simulink model "CF016A_GmVehSpdArbn"  (R2013b)
settings: Solver=FixedStepDiscrete  SolverMode=SingleTasking  StartTime=0.0  StopTime=1  FixedStep=0.002  RelTol=1e-3
undefined symbols (not defined in the file): DIAGCSTRTUPDLY_CNT_U32, NODEBSTEP_CNT_U16, NtcNr1, NtcSts1, VEHSPDMAX_KPH_F32
libraries: simulink x8, NxtrMax x7, NxtrMin x3, NxtrLim x3
(part 5 of 5)

== system CF016A_GmVehSpdArbn/GmVehSpdArbn/GmVehSpdArbnPer1/LeDrvnVld/Set_LeDrvnVld_False ==
  Action Port : ActionPort  ActionType=then
  Constant2 : Constant  Value=false  OutDataTypeStr=boolean
      settings: AttributesFormatString=%<OutDataTypeStr>
  CopyRight2 : Subsystem  Description=|  mask(Copyright Information){none=on}
      | Copyright info block.                                               
      |                                                                     
      | Place copyright information at the top of every subsystem in design.
      mask prompts: none "No parameters"
      mask help: Place copyright information at the top of every subsystem in design.
      mask Display:
      | NxtrConf = 'Nexteer Confidential';
      | 
      | sys = bdroot; %handle for the current model ("system")
      | first = get_param(sys,'Created');
      | if(isempty(first))
      |     first = datestr(now,'yyyy');
      | else
      |     first = first(end-3:end);  %year is last four digits
      | end
      | 
      | last = get_param(sys,'LastModifiedDate');
      | if isempty(last)
      |     last = datestr(now,'yyyy');
      | else
      |     last = last(end-3:end);
      | end
      | 
      | if strcmp(first,last)
      |     fprintf('%s -- Copyright %s Nexteer',NxtrConf,first)
      | else
      |     fprintf('%s -- %s%s- %s Nexteer',NxtrConf,char(169),first,last)
      | end
  LeDrvnVld : Outport
  wires:
  Constant2/1 -> LeDrvnVld/1

== system CF016A_GmVehSpdArbn/GmVehSpdArbn/GmVehSpdArbnPer1/LeDrvnVld/Set_LeDrvnVld_True ==
  Action Port : ActionPort  ActionType=else
  Constant2 : Constant  Value=true  OutDataTypeStr=boolean
      settings: AttributesFormatString=%<OutDataTypeStr>
  CopyRight2 : Subsystem  Description=|  mask(Copyright Information){none=on}
      | Copyright info block.                                               
      |                                                                     
      | Place copyright information at the top of every subsystem in design.
      mask prompts: none "No parameters"
      mask help: Place copyright information at the top of every subsystem in design.
      mask Display:
      | NxtrConf = 'Nexteer Confidential';
      | 
      | sys = bdroot; %handle for the current model ("system")
      | first = get_param(sys,'Created');
      | if(isempty(first))
      |     first = datestr(now,'yyyy');
      | else
      |     first = first(end-3:end);  %year is last four digits
      | end
      | 
      | last = get_param(sys,'LastModifiedDate');
      | if isempty(last)
      |     last = datestr(now,'yyyy');
      | else
      |     last = last(end-3:end);
      | end
      | 
      | if strcmp(first,last)
      |     fprintf('%s -- Copyright %s Nexteer',NxtrConf,first)
      | else
      |     fprintf('%s -- %s%s- %s Nexteer',NxtrConf,char(169),first,last)
      | end
  LeDrvnVld : Outport
  wires:
  Constant2/1 -> LeDrvnVld/1

== system CF016A_GmVehSpdArbn/GmVehSpdArbn/GmVehSpdArbnPer1/LeNonDrvnVld/CopyRight2 ==

== system CF016A_GmVehSpdArbn/GmVehSpdArbn/GmVehSpdArbnPer1/LeNonDrvnVld/Set_LeNonDrvnVld_False ==
  Action Port : ActionPort  ActionType=then
  Constant2 : Constant  Value=false  OutDataTypeStr=boolean
      settings: AttributesFormatString=%<OutDataTypeStr>
  CopyRight2 : Subsystem  Description=|  mask(Copyright Information){none=on}
      | Copyright info block.                                               
      |                                                                     
      | Place copyright information at the top of every subsystem in design.
      mask prompts: none "No parameters"
      mask help: Place copyright information at the top of every subsystem in design.
      mask Display:
      | NxtrConf = 'Nexteer Confidential';
      | 
      | sys = bdroot; %handle for the current model ("system")
      | first = get_param(sys,'Created');
      | if(isempty(first))
      |     first = datestr(now,'yyyy');
      | else
      |     first = first(end-3:end);  %year is last four digits
      | end
      | 
      | last = get_param(sys,'LastModifiedDate');
      | if isempty(last)
      |     last = datestr(now,'yyyy');
      | else
      |     last = last(end-3:end);
      | end
      | 
      | if strcmp(first,last)
      |     fprintf('%s -- Copyright %s Nexteer',NxtrConf,first)
      | else
      |     fprintf('%s -- %s%s- %s Nexteer',NxtrConf,char(169),first,last)
      | end
  LeNonDrvnVld : Outport
  wires:
  Constant2/1 -> LeNonDrvnVld/1

== system CF016A_GmVehSpdArbn/GmVehSpdArbn/GmVehSpdArbnPer1/LeNonDrvnVld/Set_LeNonDrvnVld_True ==
  Action Port : ActionPort  ActionType=else
  Constant2 : Constant  Value=true  OutDataTypeStr=boolean
      settings: AttributesFormatString=%<OutDataTypeStr>
  CopyRight2 : Subsystem  Description=|  mask(Copyright Information){none=on}
      | Copyright info block.                                               
      |                                                                     
      | Place copyright information at the top of every subsystem in design.
      mask prompts: none "No parameters"
      mask help: Place copyright information at the top of every subsystem in design.
      mask Display:
      | NxtrConf = 'Nexteer Confidential';
      | 
      | sys = bdroot; %handle for the current model ("system")
      | first = get_param(sys,'Created');
      | if(isempty(first))
      |     first = datestr(now,'yyyy');
      | else
      |     first = first(end-3:end);  %year is last four digits
      | end
      | 
      | last = get_param(sys,'LastModifiedDate');
      | if isempty(last)
      |     last = datestr(now,'yyyy');
      | else
      |     last = last(end-3:end);
      | end
      | 
      | if strcmp(first,last)
      |     fprintf('%s -- Copyright %s Nexteer',NxtrConf,first)
      | else
      |     fprintf('%s -- %s%s- %s Nexteer',NxtrConf,char(169),first,last)
      | end
  LeNonDrvnVld : Outport
  wires:
  Constant2/1 -> LeNonDrvnVld/1

== system CF016A_GmVehSpdArbn/GmVehSpdArbn/GmVehSpdArbnPer1/RiDrvnVld/CopyRight2 ==

== system CF016A_GmVehSpdArbn/GmVehSpdArbn/GmVehSpdArbnPer1/RiDrvnVld/Set_RiDrvnVld_False ==
  Action Port : ActionPort  ActionType=then
  Constant2 : Constant  Value=false  OutDataTypeStr=boolean
      settings: AttributesFormatString=%<OutDataTypeStr>
  CopyRight2 : Subsystem  Description=|  mask(Copyright Information){none=on}
      | Copyright info block.                                               
      |                                                                     
      | Place copyright information at the top of every subsystem in design.
      mask prompts: none "No parameters"
      mask help: Place copyright information at the top of every subsystem in design.
      mask Display:
      | NxtrConf = 'Nexteer Confidential';
      | 
      | sys = bdroot; %handle for the current model ("system")
      | first = get_param(sys,'Created');
      | if(isempty(first))
      |     first = datestr(now,'yyyy');
      | else
      |     first = first(end-3:end);  %year is last four digits
      | end
      | 
      | last = get_param(sys,'LastModifiedDate');
      | if isempty(last)
      |     last = datestr(now,'yyyy');
      | else
      |     last = last(end-3:end);
      | end
      | 
      | if strcmp(first,last)
      |     fprintf('%s -- Copyright %s Nexteer',NxtrConf,first)
      | else
      |     fprintf('%s -- %s%s- %s Nexteer',NxtrConf,char(169),first,last)
      | end
  RiDrvnVld : Outport
  wires:
  Constant2/1 -> RiDrvnVld/1

== system CF016A_GmVehSpdArbn/GmVehSpdArbn/GmVehSpdArbnPer1/RiDrvnVld/Set_RiDrvnVld_True ==
  Action Port : ActionPort  ActionType=else
  Constant2 : Constant  Value=true  OutDataTypeStr=boolean
      settings: AttributesFormatString=%<OutDataTypeStr>
  CopyRight2 : Subsystem  Description=|  mask(Copyright Information){none=on}
      | Copyright info block.                                               
      |                                                                     
      | Place copyright information at the top of every subsystem in design.
      mask prompts: none "No parameters"
      mask help: Place copyright information at the top of every subsystem in design.
      mask Display:
      | NxtrConf = 'Nexteer Confidential';
      | 
      | sys = bdroot; %handle for the current model ("system")
      | first = get_param(sys,'Created');
      | if(isempty(first))
      |     first = datestr(now,'yyyy');
      | else
      |     first = first(end-3:end);  %year is last four digits
      | end
      | 
      | last = get_param(sys,'LastModifiedDate');
      | if isempty(last)
      |     last = datestr(now,'yyyy');
      | else
      |     last = last(end-3:end);
      | end
      | 
      | if strcmp(first,last)
      |     fprintf('%s -- Copyright %s Nexteer',NxtrConf,first)
      | else
      |     fprintf('%s -- %s%s- %s Nexteer',NxtrConf,char(169),first,last)
      | end
  RiDrvnVld : Outport
  wires:
  Constant2/1 -> RiDrvnVld/1

== system CF016A_GmVehSpdArbn/GmVehSpdArbn/GmVehSpdArbnPer1/RiNonDrvnVld/CopyRight2 ==

== system CF016A_GmVehSpdArbn/GmVehSpdArbn/GmVehSpdArbnPer1/RiNonDrvnVld/Set_RiNonDrvnVld_False ==
  Action Port : ActionPort  ActionType=then
  Constant2 : Constant  Value=false  OutDataTypeStr=boolean
      settings: AttributesFormatString=%<OutDataTypeStr>
  CopyRight2 : Subsystem  Description=|  mask(Copyright Information){none=on}
      | Copyright info block.                                               
      |                                                                     
      | Place copyright information at the top of every subsystem in design.
      mask prompts: none "No parameters"
      mask help: Place copyright information at the top of every subsystem in design.
      mask Display:
      | NxtrConf = 'Nexteer Confidential';
      | 
      | sys = bdroot; %handle for the current model ("system")
      | first = get_param(sys,'Created');
      | if(isempty(first))
      |     first = datestr(now,'yyyy');
      | else
      |     first = first(end-3:end);  %year is last four digits
      | end
      | 
      | last = get_param(sys,'LastModifiedDate');
      | if isempty(last)
      |     last = datestr(now,'yyyy');
      | else
      |     last = last(end-3:end);
      | end
      | 
      | if strcmp(first,last)
      |     fprintf('%s -- Copyright %s Nexteer',NxtrConf,first)
      | else
      |     fprintf('%s -- %s%s- %s Nexteer',NxtrConf,char(169),first,last)
      | end
  RiNonDrvnVld : Outport
  wires:
  Constant2/1 -> RiNonDrvnVld/1

== system CF016A_GmVehSpdArbn/GmVehSpdArbn/GmVehSpdArbnPer1/RiNonDrvnVld/Set_RiNonDrvnVld_True ==
  Action Port : ActionPort  ActionType=else
  Constant2 : Constant  Value=true  OutDataTypeStr=boolean
      settings: AttributesFormatString=%<OutDataTypeStr>
  CopyRight2 : Subsystem  Description=|  mask(Copyright Information){none=on}
      | Copyright info block.                                               
      |                                                                     
      | Place copyright information at the top of every subsystem in design.
      mask prompts: none "No parameters"
      mask help: Place copyright information at the top of every subsystem in design.
      mask Display:
      | NxtrConf = 'Nexteer Confidential';
      | 
      | sys = bdroot; %handle for the current model ("system")
      | first = get_param(sys,'Created');
      | if(isempty(first))
      |     first = datestr(now,'yyyy');
      | else
      |     first = first(end-3:end);  %year is last four digits
      | end
      | 
      | last = get_param(sys,'LastModifiedDate');
      | if isempty(last)
      |     last = datestr(now,'yyyy');
      | else
      |     last = last(end-3:end);
      | end
      | 
      | if strcmp(first,last)
      |     fprintf('%s -- Copyright %s Nexteer',NxtrConf,first)
      | else
      |     fprintf('%s -- %s%s- %s Nexteer',NxtrConf,char(169),first,last)
      | end
  RiNonDrvnVld : Outport
  wires:
  Constant2/1 -> RiNonDrvnVld/1

== system CF016A_GmVehSpdArbn/GmVehSpdArbn/GmVehSpdArbnPer1/VehSpdMaxSecur_Invld/CopyRight2 ==

== system CF016A_GmVehSpdArbn/GmVehSpdArbn/GmVehSpdArbnPer1/VehSpdMinSecur_Invld/CopyRight2 ==

== system CF016A_GmVehSpdArbn/GmVehSpdArbn/GmVehSpdArbnPer1/ArbdFalseAndSnsrFalse_NTCFaild/NTC_0x0E0/SetNtcSts ==
  NtcNr : Inport
  NtcStInfo : Inport  Port=2
  NtcSts : Inport  Port=3
  DebStep : Inport  Port=4
  CopyRight2 : Subsystem  Description=|  mask(Copyright Information){none=on}
      | Copyright info block.                                               
      |                                                                     
      | Place copyright information at the top of every subsystem in design.
      mask prompts: none "No parameters"
      mask help: Place copyright information at the top of every subsystem in design.
      mask Display:
      | NxtrConf = 'Nexteer Confidential';
      | 
      | sys = bdroot; %handle for the current model ("system")
      | first = get_param(sys,'Created');
      | first = first(end-3:end);  %year is last four digits
      | 
      | last = get_param(sys,'LastModifiedDate');
      | if isempty(last)
      |     last = datestr(now,'yyyy');
      | else
      |     last = last(end-3:end);
      | end
      | 
      | if strcmp(first,last)
      |     fprintf('%s -- Copyright %s Nexteer',NxtrConf,first)
      | else
      |     fprintf('%s -- %s%s- %s Nexteer',NxtrConf,char(169),first,last)
      | end
  Data Store Write3 : DataStoreWrite  DataStoreName=NonSecurVehSpdInvld
  Terminator : Terminator
  Terminator1 : Terminator
  Terminator2 : Terminator
  wires:
  NtcStInfo/1 -> Terminator1/1
  NtcNr/1 -> Terminator/1
  NtcSts/1 -> Data Store Write3/1
  DebStep/1 -> Terminator2/1

== system CF016A_GmVehSpdArbn/GmVehSpdArbn/GmVehSpdArbnPer1/ArbdFalseAndSnsrTrue_NTCPassd/NTC_0x0E0/SetNtcSts ==
  NtcNr : Inport
  NtcStInfo : Inport  Port=2
  NtcSts : Inport  Port=3
  DebStep : Inport  Port=4
  CopyRight2 : Subsystem  Description=|  mask(Copyright Information){none=on}
      | Copyright info block.                                               
      |                                                                     
      | Place copyright information at the top of every subsystem in design.
      mask prompts: none "No parameters"
      mask help: Place copyright information at the top of every subsystem in design.
      mask Display:
      | NxtrConf = 'Nexteer Confidential';
      | 
      | sys = bdroot; %handle for the current model ("system")
      | first = get_param(sys,'Created');
      | first = first(end-3:end);  %year is last four digits
      | 
      | last = get_param(sys,'LastModifiedDate');
      | if isempty(last)
      |     last = datestr(now,'yyyy');
      | else
      |     last = last(end-3:end);
      | end
      | 
      | if strcmp(first,last)
      |     fprintf('%s -- Copyright %s Nexteer',NxtrConf,first)
      | else
      |     fprintf('%s -- %s%s- %s Nexteer',NxtrConf,char(169),first,last)
      | end
  Data Store Write3 : DataStoreWrite  DataStoreName=NonSecurVehSpdInvld
  Terminator : Terminator
  Terminator1 : Terminator
  Terminator2 : Terminator
  wires:
  DebStep/1 -> Terminator2/1
  NtcSts/1 -> Data Store Write3/1
  NtcNr/1 -> Terminator/1
  NtcStInfo/1 -> Terminator1/1

== system CF016A_GmVehSpdArbn/GmVehSpdArbn/GmVehSpdArbnPer1/ArbdTrueAndSnsrTrue_NTCPassd/NTC_0x0E0/SetNtcSts ==
  NtcNr : Inport
  NtcStInfo : Inport  Port=2
  NtcSts : Inport  Port=3
  DebStep : Inport  Port=4
  CopyRight2 : Subsystem  Description=|  mask(Copyright Information){none=on}
      | Copyright info block.                                               
      |                                                                     
      | Place copyright information at the top of every subsystem in design.
      mask prompts: none "No parameters"
      mask help: Place copyright information at the top of every subsystem in design.
      mask Display:
      | NxtrConf = 'Nexteer Confidential';
      | 
      | sys = bdroot; %handle for the current model ("system")
      | first = get_param(sys,'Created');
      | first = first(end-3:end);  %year is last four digits
      | 
      | last = get_param(sys,'LastModifiedDate');
      | if isempty(last)
      |     last = datestr(now,'yyyy');
      | else
      |     last = last(end-3:end);
      | end
      | 
      | if strcmp(first,last)
      |     fprintf('%s -- Copyright %s Nexteer',NxtrConf,first)
      | else
      |     fprintf('%s -- %s%s- %s Nexteer',NxtrConf,char(169),first,last)
      | end
  Data Store Write3 : DataStoreWrite  DataStoreName=NonSecurVehSpdInvld
  Terminator : Terminator
  Terminator1 : Terminator
  Terminator2 : Terminator
  wires:
  DebStep/1 -> Terminator2/1
  NtcSts/1 -> Data Store Write3/1
  NtcNr/1 -> Terminator/1
  NtcStInfo/1 -> Terminator1/1

== system CF016A_GmVehSpdArbn/GmVehSpdArbn/GmVehSpdArbnPer1/Calc_NTCIdleTi/GetTiSpan100MicroSec32bit/CopyRight2 ==

== system CF016A_GmVehSpdArbn/GmVehSpdArbn/GmVehSpdArbnPer1/Calc_NTCIdleTi/GetTiSpan100MicroSec32bit/Nowrapping ==
  new : Inport
  ref : Inport  Port=2
  Action Port : ActionPort  ActionType=then
  CopyRight2 : Subsystem  Description=|  mask(Copyright Information){none=on}
      | Copyright info block.                                               
      |                                                                     
      | Place copyright information at the top of every subsystem in design.
      mask prompts: none "No parameters"
      mask help: Place copyright information at the top of every subsystem in design.
      mask Display:
      | NxtrConf = 'Nexteer Confidential';
      | 
      | sys = bdroot; %handle for the current model ("system")
      | first = get_param(sys,'Created');
      | if(isempty(first))
      |     first = datestr(now,'yyyy');
      | else
      |     first = first(end-3:end);  %year is last four digits
      | end
      | 
      | last = get_param(sys,'LastModifiedDate');
      | if isempty(last)
      |     last = datestr(now,'yyyy');
      | else
      |     last = last(end-3:end);
      | end
      | 
      | if strcmp(first,last)
      |     fprintf('%s -- Copyright %s Nexteer',NxtrConf,first)
      | else
      |     fprintf('%s -- %s%s- %s Nexteer',NxtrConf,char(169),first,last)
      | end
  Subtract1 : Sum  Inputs=+-
  Out1 : Outport
  wires:
  Subtract1/1 -> Out1/1
  new/1 -> Subtract1/1
  ref/1 -> Subtract1/2

== system CF016A_GmVehSpdArbn/GmVehSpdArbn/GmVehSpdArbnPer1/Calc_NTCIdleTi/GetTiSpan100MicroSec32bit/Wrapping ==
  new : Inport
  ref : Inport  Port=2
  Action Port : ActionPort  ActionType=else
  CopyRight2 : Subsystem  Description=|  mask(Copyright Information){none=on}
      | Copyright info block.                                               
      |                                                                     
      | Place copyright information at the top of every subsystem in design.
      mask prompts: none "No parameters"
      mask help: Place copyright information at the top of every subsystem in design.
      mask Display:
      | NxtrConf = 'Nexteer Confidential';
      | 
      | sys = bdroot; %handle for the current model ("system")
      | first = get_param(sys,'Created');
      | if(isempty(first))
      |     first = datestr(now,'yyyy');
      | else
      |     first = first(end-3:end);  %year is last four digits
      | end
      | 
      | last = get_param(sys,'LastModifiedDate');
      | if isempty(last)
      |     last = datestr(now,'yyyy');
      | else
      |     last = last(end-3:end);
      | end
      | 
      | if strcmp(first,last)
      |     fprintf('%s -- Copyright %s Nexteer',NxtrConf,first)
      | else
      |     fprintf('%s -- %s%s- %s Nexteer',NxtrConf,char(169),first,last)
      | end
  Max Counts : Constant  Value=2^32-1  OutDataTypeStr=uint32
  Subtract1 : Sum  Inputs=+-+
  Out1 : Outport
  wires:
  Subtract1/1 -> Out1/1
  Max Counts/1 -> Subtract1/1
  ref/1 -> Subtract1/2
  new/1 -> Subtract1/3

== system CF016A_GmVehSpdArbn/GmVehSpdArbn/GmVehSpdArbnPer1/Calc_SpdArbd/Calc_VehSpdArbd/CopyRight2 ==

== system CF016A_GmVehSpdArbn/GmVehSpdArbn/GmVehSpdArbnPer1/Calc_SpdArbd/Pass_TmpSpdArbd/CopyRight2 ==

== system CF016A_GmVehSpdArbn/GmVehSpdArbn/GmVehSpdArbnPer1/Calc_TmpSpdArbd_SpdArbdCnt/CalcSumCnt/CopyRight2 ==

== system CF016A_GmVehSpdArbn/GmVehSpdArbn/GmVehSpdArbnPer1/Calc_TmpSpdArbd_SpdArbdCnt/CalcSumCnt_1/CopyRight2 ==

== system CF016A_GmVehSpdArbn/GmVehSpdArbn/GmVehSpdArbnPer1/Calc_TmpSpdArbd_SpdArbdCnt/CalcSumCnt_2/CopyRight2 ==

== system CF016A_GmVehSpdArbn/GmVehSpdArbn/GmVehSpdArbnPer1/Calc_TmpSpdArbd_SpdArbdCnt/CalcSumCnt_3/CopyRight2 ==

== system CF016A_GmVehSpdArbn/GmVehSpdArbn/GmVehSpdArbnPer1/Calc_TmpSpdArbd_SpdArbdCnt/Pass_0s/CopyRight2 ==

== system CF016A_GmVehSpdArbn/GmVehSpdArbn/GmVehSpdArbnPer1/Calc_TmpSpdArbd_SpdArbdCnt/Pass_TmpSpdArbd_SpdArbdCnt_1/CopyRight2 ==

== system CF016A_GmVehSpdArbn/GmVehSpdArbn/GmVehSpdArbnPer1/Calc_TmpSpdArbd_SpdArbdCnt/Pass_TmpSpdArbd_SpdArbdCnt_2/CopyRight2 ==

== system CF016A_GmVehSpdArbn/GmVehSpdArbn/GmVehSpdArbnPer1/Calc_TmpSpdArbd_SpdArbdCnt/Pass_TmpSpdArbd_SpdArbdCnt_3/CopyRight2 ==

== system CF016A_GmVehSpdArbn/GmVehSpdArbn/GmVehSpdArbnPer1/Calc_VehSpdMaxSecur/Calc_VehSpdMaxSecur/CopyRight2 ==

== system CF016A_GmVehSpdArbn/GmVehSpdArbn/GmVehSpdArbnPer1/Calc_VehSpdMaxSecur/Calc_VehSpdMaxSecur1/CopyRight2 ==

== system CF016A_GmVehSpdArbn/GmVehSpdArbn/GmVehSpdArbnPer1/Calc_VehSpdMaxSecur/Calc_VehSpdMaxSecur2/CopyRight2 ==

== system CF016A_GmVehSpdArbn/GmVehSpdArbn/GmVehSpdArbnPer1/Calc_VehSpdMaxSecur/Calc_VehSpdMaxSecur3/CopyRight2 ==

== system CF016A_GmVehSpdArbn/GmVehSpdArbn/GmVehSpdArbnPer1/Calc_VehSpdMaxSecur/Pass_0/CopyRight2 ==

== system CF016A_GmVehSpdArbn/GmVehSpdArbn/GmVehSpdArbnPer1/Calc_VehSpdMaxSecur/Pass_VehSpdMaxSecur1/CopyRight2 ==

== system CF016A_GmVehSpdArbn/GmVehSpdArbn/GmVehSpdArbnPer1/Calc_VehSpdMaxSecur/Pass_VehSpdMaxSecur2/CopyRight2 ==

== system CF016A_GmVehSpdArbn/GmVehSpdArbn/GmVehSpdArbnPer1/Calc_VehSpdMaxSecur/Pass_VehSpdMaxSecur3/CopyRight2 ==

== system CF016A_GmVehSpdArbn/GmVehSpdArbn/GmVehSpdArbnPer1/Calc_VehSpdMinSecurVld/Get_Min/CopyRight2 ==

== system CF016A_GmVehSpdArbn/GmVehSpdArbn/GmVehSpdArbnPer1/Calc_VehSpdMinSecurVld/Min_LeNonDrvnBusHiSpd_LeNonDrvnBusChassisExp/CopyRight2 ==

== system CF016A_GmVehSpdArbn/GmVehSpdArbn/GmVehSpdArbnPer1/Calc_VehSpdMinSecurVld/Pass_VehSpdMinSecur/CopyRight2 ==

== system CF016A_GmVehSpdArbn/GmVehSpdArbn/GmVehSpdArbnPer1/Calc_VehSpdMinSecurVld/Set_VehSpdMinSecur_Max/CopyRight2 ==

== system CF016A_GmVehSpdArbn/GmVehSpdArbn/GmVehSpdArbnPer1/LeDrvnVld/Set_LeDrvnVld_False/CopyRight2 ==

== system CF016A_GmVehSpdArbn/GmVehSpdArbn/GmVehSpdArbnPer1/LeDrvnVld/Set_LeDrvnVld_True/CopyRight2 ==

== system CF016A_GmVehSpdArbn/GmVehSpdArbn/GmVehSpdArbnPer1/LeNonDrvnVld/Set_LeNonDrvnVld_False/CopyRight2 ==

== system CF016A_GmVehSpdArbn/GmVehSpdArbn/GmVehSpdArbnPer1/LeNonDrvnVld/Set_LeNonDrvnVld_True/CopyRight2 ==

== system CF016A_GmVehSpdArbn/GmVehSpdArbn/GmVehSpdArbnPer1/RiDrvnVld/Set_RiDrvnVld_False/CopyRight2 ==

== system CF016A_GmVehSpdArbn/GmVehSpdArbn/GmVehSpdArbnPer1/RiDrvnVld/Set_RiDrvnVld_True/CopyRight2 ==

== system CF016A_GmVehSpdArbn/GmVehSpdArbn/GmVehSpdArbnPer1/RiNonDrvnVld/Set_RiNonDrvnVld_False/CopyRight2 ==

== system CF016A_GmVehSpdArbn/GmVehSpdArbn/GmVehSpdArbnPer1/RiNonDrvnVld/Set_RiNonDrvnVld_True/CopyRight2 ==

== system CF016A_GmVehSpdArbn/GmVehSpdArbn/GmVehSpdArbnPer1/ArbdFalseAndSnsrFalse_NTCFaild/NTC_0x0E0/SetNtcSts/CopyRight2 ==

== system CF016A_GmVehSpdArbn/GmVehSpdArbn/GmVehSpdArbnPer1/ArbdFalseAndSnsrTrue_NTCPassd/NTC_0x0E0/SetNtcSts/CopyRight2 ==

== system CF016A_GmVehSpdArbn/GmVehSpdArbn/GmVehSpdArbnPer1/ArbdTrueAndSnsrTrue_NTCPassd/NTC_0x0E0/SetNtcSts/CopyRight2 ==

== system CF016A_GmVehSpdArbn/GmVehSpdArbn/GmVehSpdArbnPer1/Calc_NTCIdleTi/GetTiSpan100MicroSec32bit/Nowrapping/CopyRight2 ==

== system CF016A_GmVehSpdArbn/GmVehSpdArbn/GmVehSpdArbnPer1/Calc_NTCIdleTi/GetTiSpan100MicroSec32bit/Wrapping/CopyRight2 ==
